simulink model "testCoriolisAndMassMatrix"  (R2020a)
settings: Solver=VariableStepAuto  StartTime=0.0  StopTime=10000  RelTol=1e-3
settings Model: Creator=iiticublap041  LastModifiedBy=iiticublap041

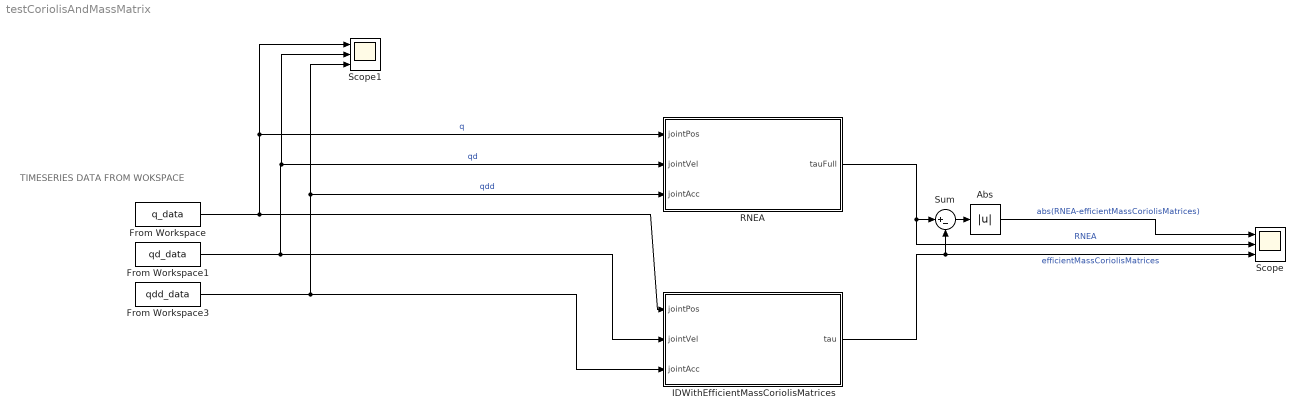
== system testCoriolisAndMassMatrix ==
  note: TIMESERIES DATA FROM WOKSPACE
  Abs : Abs
  From Workspace : FromWorkspace  VariableName=q_data
  From Workspace1 : FromWorkspace  VariableName=qd_data
  From Workspace3 : FromWorkspace  VariableName=qdd_data
  IDWithEfficientMassCoriolisMatrices : MATLAB Function  TreatAsAtomicUnit=on
  RNEA : MATLAB Function  TreatAsAtomicUnit=on
  Scope : Scope  NumInputPorts=3
  Scope1 : Scope  NumInputPorts=3
  Sum : Sum  Inputs=|+-
  wires:
  From Workspace/1 -> IDWithEfficientMassCoriolisMatrices/1(jointPos), RNEA/1(jointPos), Scope1/1  "q"
  From Workspace1/1 -> IDWithEfficientMassCoriolisMatrices/2(jointVel), Scope1/2, RNEA/2(jointVel)  "qd"
  From Workspace3/1 -> IDWithEfficientMassCoriolisMatrices/3(jointAcc), Scope1/3, RNEA/3(jointAcc)  "qdd"
  RNEA/1(tauFull) -> Scope/2, Sum/1  "RNEA"
  IDWithEfficientMassCoriolisMatrices/1(tau) -> Scope/3, Sum/2  "efficientMassCoriolisMatrices"
  Sum/1 -> Abs/1
  Abs/1 -> Scope/1  "abs(RNEA-efficientMassCoriolisMatrices)"

== matlab function testCoriolisAndMassMatrix/IDWithEfficientMassCoriolisMatrices ==
  data: jointPos input; jointVel input; tau output; jointAcc input
function tau = computeInverseDynamics(jointPos,jointVel,jointAcc)

% Zero external forces
F_ext = 0;
% TODO: do not hard code gravity 
g = [0;0;-9.81];

% Use computeMassMatrix mex function
coder.extrinsic('computeMassMatrix');
M = computeMassMatrix('computeMassMatrix',jointPos);

% Use computeCoriolisMatrix mex function
coder.extrinsic('computeCoriolisMatrix');
C = computeCoriolisMatrix('computeCoriolisMatrix',jointPos,jointVel);

% Use rnea mex function to compute gravity torques
coder.extrinsic('rnea');
tau_g = rnea('rnea',jointPos,0,0,g,0);

% Assign the output to a vaiable of known type.
% See https://www.mathworks.com/help/simulink/ug/calling-matlab-functions.html#bq1h2z9-47
MFull = zeros(max(size(jointPos)));
CFull = zeros(max(size(jointPos)));
tau_gFull = zeros(max(size(jointPos)),1);
MFull = full(M);
CFull = full(C);
tau_gFull = full(tau_g);

tau = MFull*jointAcc + CFull*jointVel + tau_gFull;
end

== matlab function testCoriolisAndMassMatrix/RNEA ==
  data: jointPos input; jointVel input; tauFull output; jointAcc input
function tauFull = RNEA(jointPos,jointVel,jointAcc)

% Zero external forces
F_ext = 0;
% TODO: do not hard code gravity 
g = [0;0;-9.81];
% Use rnea mex function
coder.extrinsic('rnea');
tau = rnea('rnea',jointPos,jointVel,jointAcc,g,F_ext);
% Assign the output to a vaiable of known type.
% See https://www.mathworks.com/help/simulink/ug/calling-matlab-functions.html#bq1h2z9-47
tauFull = zeros(max(size(jointPos)),1);
tauFull = full(tau);
end
